simulink model "FAST"  (R2017b)
settings: Solver=FixedStepAuto  StartTime=0.0  StopTime=TMax  FixedStep=DT  RelTol=1e-3
values from neighbouring files (symbols this model uses):
  CertificationSettings = handles.CertificationSettings    [Certification.m]
  Control = handles.Control    [Certification.m]    (also in Linearization.m)
  dLP = ss(c2d(LP, Control.DT))    [ControllerDesign.m]
  dLP_IPC = ss(c2d(LP_IPC, Control.DT))    [ControllerDesign.m]
  dNotch = ss(c2d(Notch, Control.DT))    [ControllerDesign.m]
  Drivetrain = handles.Drivetrain    [Certification.m]    (also in Linearization.m)
  P_InitAngle = Control.Pitch.Max    [Certification.m]
  RPM_Init = 0    [Certification.m]
undefined symbols (not defined in the file or in its folder): AziPhase_offset_rev_1P, AziPhase_offset_rev_2P, DisableIPC_1P, DisableIPC_2P, DiscIntNeverNeededParam, OutList, strmatch, T_GenSpeedInit
libraries: simulink x5
(part 1 of 2)
settings Model: ExtModeTrigMode=oneshot  ExtModeArmWhenConnect=off  Creator=Hazim Namik  LastModifiedBy=sebastiaanmuld
settings DataIOCC: LimitDataPoints=on  SaveFormat=Array
settings OptimizationCC: BlockReduction=off  BooleanDataType=off  LifeSpan=inf
settings DebuggingCC: SaveWithParameterizedLinksMsg=none  UnderspecifiedInitializationDetection=Classic  MergeDetectMultiDrivingBlocksExec=none  SignalResolutionControl=TryResolveAllWithWarning  SFUnexpectedBacktrackingDiag=warning  SFNoUnconditionalDefaultTransitionDiag=warning  SFExecutionAtInitializationDiag=none
settings HardwareCC: ProdBitPerPointer=32  ProdBitPerSizeT=32  ProdBitPerPtrDiffT=32  ProdLargestAtomicFloat=None  ProdIntDivRoundTo=Undefined  ProdEndianess=Unspecified  ProdWordSize=32  ProdHWDeviceType=32-bit Generic  TargetUnknown=on
settings ModelReferenceCC: PropagateSignalLabelsOutOfModel=off
settings CodeAppCC: StateflowObjectComments=on
settings GRTTargetCC: TargetLangStandard=C89/C90 (ANSI)  GeneratePreprocessorConditionals=Disable all
settings ConfigComp: CovMetricSettings=dw  CovHtmlReporting=on  CovSaveCumulativeToWorkspaceVar=on  CovSaveSingleToWorkspaceVar=on  CovExternalEMLEnable=off

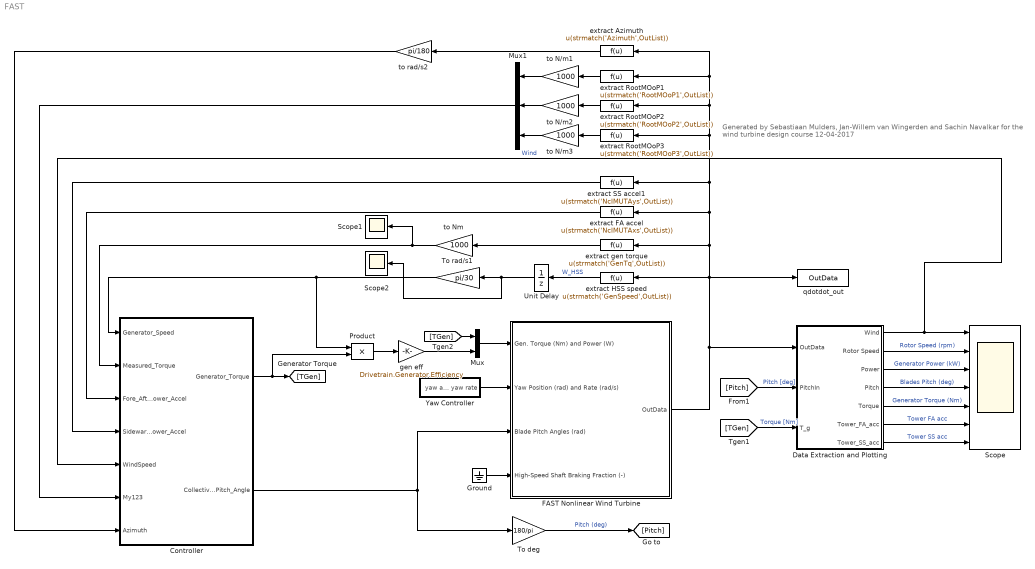
== system FAST ==
  note: Generated by Sebastiaan Mulders, Jan-Willem van Wingerden and Sachin Navalkar
      | for the wind turbine design course 12-04-2017
  Controller : Subsystem
  Data Extraction and Plotting : Subsystem
  FAST Nonlinear Wind Turbine : Subsystem  mask(FAST Nonlinear Wind Turbine){}
      mask help: This block contains the FAST S-Function.
      mask init:
      | clear FAST_SFunc
  Ground : Ground
  Mux : Mux  Inputs=2
  Mux1 : Mux  Inputs=3
  Product : Product  RndMeth=Zero
  Scope : Scope  NumInputPorts=7
      settings: Tag=Scope
  Scope1 : Scope
  Scope2 : Scope
  To deg : Gain  Gain=180/pi
  To rad/s1 : Gain  Gain=pi/30
  Unit Delay : UnitDelay  InitialCondition=RPM_Init*Drivetrain.Gearbox.Ratio  SampleTime=-1
  Yaw Controller : Subsystem
  extract Azimuth : Fcn  Expr=u(strmatch('Azimuth',OutList))
  extract FA accel : Fcn  Expr=u(strmatch('NcIMUTAxs',OutList))
  extract HSS speed : Fcn  Expr=u(strmatch('GenSpeed',OutList))
  extract RootMOoP1 : Fcn  Expr=u(strmatch('RootMOoP1',OutList))
  extract RootMOoP2 : Fcn  Expr=u(strmatch('RootMOoP2',OutList))
  extract RootMOoP3 : Fcn  Expr=u(strmatch('RootMOoP3',OutList))
  extract SS accel1 : Fcn  Expr=u(strmatch('NcIMUTAys',OutList))
  extract gen torque : Fcn  Expr=u(strmatch('GenTq',OutList))
  gen eff : Gain  Gain=Drivetrain.Generator.Efficiency
  qdotdot_out : ToWorkspace  VariableName=OutData  SampleTime=-1
      settings: Save2DSignal=2-D array (concatenate along first dimension)
  to N/m1 : Gain  Gain=1000
  to N/m2 : Gain  Gain=1000
  to N/m3 : Gain  Gain=1000
  to Nm : Gain  Gain=1000
  to rad/s2 : Gain  Gain=pi/180
  wires:
  Mux/1 -> FAST Nonlinear Wind Turbine/1(Gen. Torque (Nm) and Power (W))
  Yaw Controller/1(yaw and yaw rate) -> FAST Nonlinear Wind Turbine/2(Yaw Position (rad) and Rate (rad/s))
  extract HSS speed/1 -> Unit Delay/1  "W_HSS"
  To deg/1 -> [Pitch]  "Pitch (deg)"
  gen eff/1 -> Mux/2
  Product/1 -> gen eff/1
  To rad/s1/1 -> Product/1, Controller/1(Generator_Speed)
  Data Extraction and Plotting/3(Power) -> Scope/3  "Generator Power (kW)"
  [Pitch] -> Data Extraction and Plotting/2(PitchIn)  "Pitch [deg]"
  Data Extraction and Plotting/1(Wind) -> Controller/5(WindSpeed), Scope/1  "Wind"
  Data Extraction and Plotting/2(Rotor Speed) -> Scope/2  "Rotor Speed (rpm)"
  [TGen] -> Data Extraction and Plotting/3(T_g)  "Torque [Nm]"
  FAST Nonlinear Wind Turbine/1(OutData) -> extract Azimuth/1, extract RootMOoP1/1, extract RootMOoP2/1, extract RootMOoP3/1, extract SS accel1/1, extract FA accel/1, extract gen torque/1, extract HSS speed/1, qdotdot_out/1, Data Extraction and Plotting/1(OutData)
  Data Extraction and Plotting/4(Pitch) -> Scope/4  "Blades Pitch (deg)"
  Data Extraction and Plotting/5(Torque) -> Scope/5  "Generator Torque (Nm)"
  Unit Delay/1 -> Scope2/1, To rad/s1/1
  extract gen torque/1 -> to Nm/1
  to Nm/1 -> Scope1/1, Controller/2(Measured_Torque)
  Controller/1(Generator_Torque) -> Product/2, [TGen]
  Controller/2(Collective_Pitch_Angle) -> FAST Nonlinear Wind Turbine/3(Blade Pitch Angles (rad)), To deg/1
  extract FA accel/1 -> Controller/3(Fore_Aft_Tower_Accel)
  extract SS accel1/1 -> Controller/4(Sidewards_Tower_Accel)
  Data Extraction and Plotting/6(Tower_FA_acc) -> Scope/6  "Tower FA acc"
  Data Extraction and Plotting/7(Tower_SS_acc) -> Scope/7  "Tower SS acc"
  Ground/1 -> FAST Nonlinear Wind Turbine/4(High-Speed Shaft Braking Fraction (-))
  [TGen] -> Mux/1
  extract Azimuth/1 -> to rad/s2/1
  Mux1/1 -> Controller/6(My123)
  extract RootMOoP1/1 -> to N/m1/1
  extract RootMOoP2/1 -> to N/m2/1
  extract RootMOoP3/1 -> to N/m3/1
  to rad/s2/1 -> Controller/7(Azimuth)
  to N/m1/1 -> Mux1/1
  to N/m2/1 -> Mux1/2
  to N/m3/1 -> Mux1/3

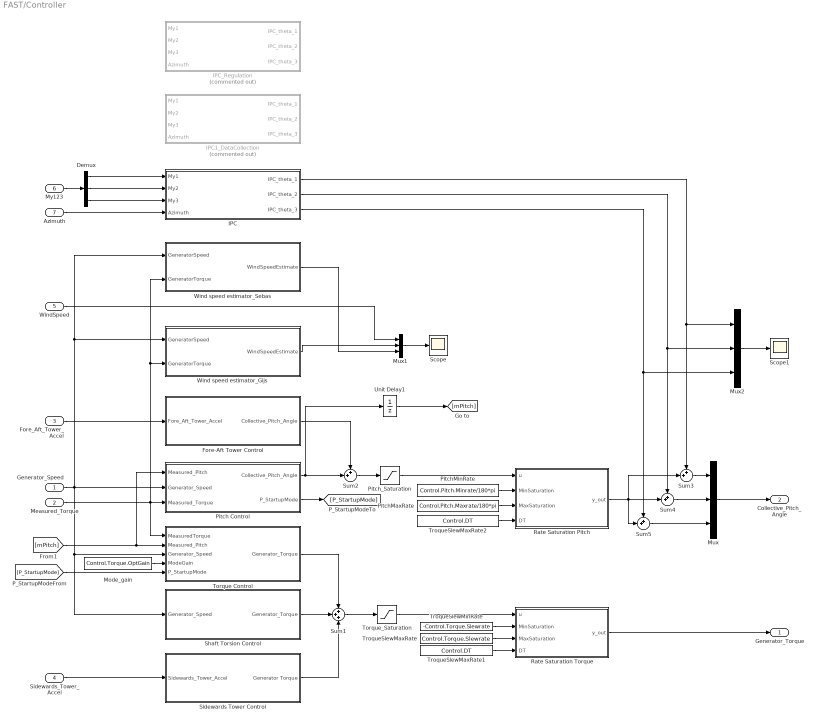
== system FAST/Controller ==
  Generator_Speed : Inport
  Measured_Torque : Inport  Port=2
  Fore_Aft_Tower_Accel : Inport  Port=3
  Sidewards_Tower_Accel : Inport  Port=4  PortDimensions=1
  WindSpeed : Inport  Port=5
  My123 : Inport  Port=6
  Azimuth : Inport  Port=7
  Demux : Demux  Outputs=3
  Fore-Aft Tower Control : Subsystem
  IPC : Subsystem
  IPC1_DataCollection : Subsystem  Commented=on
  IPC_Regulation : Subsystem  Commented=on
  Mode_gain : Constant  Value=Control.Torque.OptGain
  Mux : Mux  Inputs=3
  Mux1 : Mux  Inputs=3
  Mux2 : Mux  Inputs=3
  Pitch Control : Subsystem
  PitchMaxRate : Constant  Value=Control.Pitch.Maxrate/180*pi
  PitchMinRate : Constant  Value=Control.Pitch.Minrate/180*pi
  Pitch_Saturation : Saturate  UpperLimit=Control.Pitch.Max*pi/180  LowerLimit=Control.Pitch.Min*pi/180
  Rate Saturation Pitch : MATLAB Function  TreatAsAtomicUnit=on
  Rate Saturation Torque : MATLAB Function  TreatAsAtomicUnit=on
  Scope : Scope
  Scope1 : Scope
  Shaft Torsion Control : Subsystem
  Sidewards Tower Control : Subsystem
  Sum1 : Sum  Inputs=+++
  Sum{2..5} (4 alike) : Sum  Inputs=++|
  Torque Control : Subsystem
  Torque_Saturation : Saturate  UpperLimit=Control.Torque.Limit  LowerLimit=Control.Torque.Min
  TroqueSlewMaxRate : Constant  Value=Control.Torque.Slewrate
  TroqueSlewMaxRate1 : Constant  Value=Control.DT
  TroqueSlewMaxRate2 : Constant  Value=Control.DT
  TroqueSlewMinRate : Constant  Value=-Control.Torque.Slewrate
  Unit Delay1 : UnitDelay  InitialCondition=P_InitAngle*pi/180  SampleTime=-1
  Wind speed estimator_Gijs : Subsystem
  Wind speed estimator_Sebas : Subsystem
  Generator_Torque : Outport
  Collective_Pitch_Angle : Outport  Port=2  PortDimensions=3
  wires:
  Sidewards_Tower_Accel/1 -> Sidewards Tower Control/1(Sidewards_Tower_Accel)
  Fore_Aft_Tower_Accel/1 -> Fore-Aft Tower Control/1(Fore_Aft_Tower_Accel)
  Fore-Aft Tower Control/1(Collective_Pitch_Angle) -> Sum2/1
  Torque Control/1(Generator_Torque) -> Sum1/1
  Sidewards Tower Control/1(Generator Torque) -> Sum1/3
  [mPitch] -> Pitch Control/1(Measured_Pitch), Torque Control/2(Measured_Pitch)
  Measured_Torque/1 -> Wind speed estimator_Gijs/2(GeneratorTorque), Wind speed estimator_Sebas/2(GeneratorTorque), Torque Control/1(MeasuredTorque), Pitch Control/3(Measured_Torque)
  Shaft Torsion Control/1(Generator_Torque) -> Sum1/2
  Mode_gain/1 -> Torque Control/4(ModeGain)
  Sum1/1 -> Torque_Saturation/1
  Mux/1 -> Collective_Pitch_Angle/1
  Unit Delay1/1 -> [mPitch]
  Sum2/1 -> Pitch_Saturation/1
  Rate Saturation Pitch/1(y_out) -> Sum5/2, Sum4/2, Sum3/2
  PitchMinRate/1 -> Rate Saturation Pitch/2(MinSaturation)
  PitchMaxRate/1 -> Rate Saturation Pitch/3(MaxSaturation)
  Pitch_Saturation/1 -> Rate Saturation Pitch/1(u)
  Torque_Saturation/1 -> Rate Saturation Torque/1(u)
  TroqueSlewMinRate/1 -> Rate Saturation Torque/2(MinSaturation)
  TroqueSlewMaxRate/1 -> Rate Saturation Torque/3(MaxSaturation)
  Generator_Speed/1 -> Wind speed estimator_Sebas/1(GeneratorSpeed), Wind speed estimator_Gijs/1(GeneratorSpeed), Pitch Control/2(Generator_Speed), Torque Control/3(Generator_Speed), Shaft Torsion Control/1(Generator_Speed)
  [P_StartupMode] -> Torque Control/5(P_StartupMode)
  Pitch Control/2(P_StartupMode) -> [P_StartupMode]
  Pitch Control/1(Collective_Pitch_Angle) -> Sum2/2, Unit Delay1/1
  Rate Saturation Torque/1(y_out) -> Generator_Torque/1
  TroqueSlewMaxRate1/1 -> Rate Saturation Torque/4(DT)
  TroqueSlewMaxRate2/1 -> Rate Saturation Pitch/4(DT)
  Wind speed estimator_Gijs/1(WindSpeedEstimate) -> Mux1/2
  WindSpeed/1 -> Mux1/1
  Mux1/1 -> Scope/1
  My123/1 -> Demux/1
  Demux/1 -> IPC/1(My1)
  Demux/2 -> IPC/2(My2)
  Demux/3 -> IPC/3(My3)
  Azimuth/1 -> IPC/4(Azimuth)
  Sum3/1 -> Mux/1
  Sum4/1 -> Mux/2
  Sum5/1 -> Mux/3
  Mux2/1 -> Scope1/1
  IPC/1(IPC_theta_1) -> Mux2/1, Sum3/1
  IPC/2(IPC_theta_2) -> Mux2/2, Sum4/1
  IPC/3(IPC_theta_3) -> Sum5/1, Mux2/3
  Wind speed estimator_Sebas/1(WindSpeedEstimate) -> Mux1/3

== system FAST/Data Extraction and Plotting ==
  OutData : Inport
  PitchIn : Inport  Port=2
  T_g : Inport  Port=3
  Gain : Gain  Gain=1000
  Mux : Mux  Inputs=2
  extract Tower FA acc : Fcn  Expr=u(strmatch('NcIMUTAxs',OutList))
  extract Tower SS acc : Fcn  Expr=u(strmatch('NcIMUTAys',OutList))
  extract power : Fcn  Expr=u(strmatch('GenPwr',OutList))
  extract rotspeed : Fcn  Expr=u(strmatch('RotSpeed',OutList))
  extract w : Fcn  Expr=u(strmatch('Wind1VelX',OutList))
  extract w1 : Fcn  Expr=u(strmatch('GenTq',OutList))
  theta1 : ToWorkspace  VariableName=Tower_fa  SampleTime=-1
      settings: MaxDataPoints=Inf  Decimation=3
  theta2 : ToWorkspace  VariableName=GenPwr  SampleTime=-1
      settings: MaxDataPoints=Inf  Decimation=3
  theta3 : ToWorkspace  VariableName=wind  SampleTime=-1
      settings: MaxDataPoints=Inf  Decimation=3
  theta4 : ToWorkspace  VariableName=rotspeed  SampleTime=-1
      settings: MaxDataPoints=Inf  Decimation=3
  theta5 : ToWorkspace  VariableName=Tower_ss  SampleTime=-1
      settings: MaxDataPoints=Inf  Decimation=3
  theta6 : ToWorkspace  VariableName=pitch  SampleTime=-1
      settings: MaxDataPoints=Inf  Decimation=3
  theta7 : ToWorkspace  VariableName=Torque  SampleTime=-1
      settings: MaxDataPoints=Inf  Decimation=3
  Wind : Outport
  Rotor Speed : Outport  Port=2
  Power : Outport  Port=3
  Pitch : Outport  Port=4
  Torque : Outport  Port=5
  Tower_FA_acc : Outport  Port=6
  Tower_SS_acc : Outport  Port=7
  wires:
  extract w/1 -> Wind/1, theta3/1  "wind [m/s]"
  extract rotspeed/1 -> theta4/1, Rotor Speed/1  "rotspeed [rpm]"
  extract power/1 -> theta2/1, Power/1  "Power"
  PitchIn/1 -> theta6/1, Pitch/1
  T_g/1 -> Mux/1, theta7/1
  extract Tower FA acc/1 -> theta1/1, Tower_FA_acc/1  "Tower Fa acc"
  OutData/1 -> extract w/1, extract w1/1, extract rotspeed/1, extract Tower SS acc/1, extract Tower FA acc/1, extract power/1
  extract Tower SS acc/1 -> theta5/1, Tower_SS_acc/1  "Tower SS acc"
  extract w1/1 -> Gain/1
  Gain/1 -> Mux/2
  Mux/1 -> Torque/1

== system FAST/FAST Nonlinear Wind Turbine ==
  Gen. Torque (Nm) and Power (W) : Inport
  Yaw Position (rad) and Rate (rad/s) : Inport  Port=2
  Blade Pitch Angles (rad) : Inport  Port=3
  High-Speed Shaft Braking Fraction (-) : Inport  Port=4
  Mux1 : Mux
  S-Function : S-Function  FunctionName=FAST_SFunc  Parameters=FAST_InputFileName, TMax, 0  SFunctionDeploymentMode=off  EnableBusSupport=off
  Signal Specification1 : SignalSpecification  OutDataTypeStr=double  Dimensions=2
  Signal Specification2 : SignalSpecification  OutDataTypeStr=double  Dimensions=2
  OutData : Outport
  wires:
  Gen. Torque (Nm) and Power (W)/1 -> Signal Specification1/1
  S-Function/1 -> OutData/1
  Mux1/1 -> S-Function/1
  Blade Pitch Angles (rad)/1 -> Mux1/3
  Yaw Position (rad) and Rate (rad/s)/1 -> Signal Specification2/1
  Signal Specification1/1 -> Mux1/1
  Signal Specification2/1 -> Mux1/2
  High-Speed Shaft Braking Fraction (-)/1 -> Mux1/4

== system FAST/Yaw Controller ==
  Mux : Mux  Inputs=2
  Yaw Position : Constant  Value=0
  Yaw rate : Constant  Value=0
  yaw and yaw rate : Outport
  wires:
  Mux/1 -> yaw and yaw rate/1
  Yaw Position/1 -> Mux/1
  Yaw rate/1 -> Mux/2

== system FAST/Controller/Fore-Aft Tower Control ==
  note: Fore-Aft tower damping
  Fore_Aft_Tower_Accel : Inport
  Discrete-Time Integrator : DiscreteIntegrator  SampleTime=-1  ICPrevOutput=DiscIntNeverNeededParam  ICPrevScaledInput=DiscIntNeverNeededParam
  Gain : Gain  Gain=Control.ForeAft.Gain
  Pitch_Saturation : Saturate  UpperLimit=Control.ForeAft.MaxPitchAmplitude*pi/180  LowerLimit=-Control.ForeAft.MaxPitchAmplitude*pi/180
  Collective_Pitch_Angle : Outport
  wires:
  Fore_Aft_Tower_Accel/1 -> Discrete-Time Integrator/1
  Pitch_Saturation/1 -> Collective_Pitch_Angle/1
  Discrete-Time Integrator/1 -> Gain/1
  Gain/1 -> Pitch_Saturation/1

== system FAST/Controller/IPC ==
  My1 : Inport
  My2 : Inport  Port=2
  My3 : Inport  Port=3
  Azimuth : Inport  Port=4
  Constant : Constant
  DisableIPC : Constant  Value=DisableIPC_1P
  DisableIPC1 : Constant  Value=DisableIPC_2P
  Discrete-Time Integrator : DiscreteIntegrator  gainval=Ki_tilt_1P  ExternalReset=level  InitialConditionSetting=State (most efficient)  SampleTime=-1  LowerSaturationLimit=0  ICPrevOutput=DiscIntNeverNeededParam  ICPrevScaledInput=DiscIntNeverNeededParam
  Discrete-Time Integrator1 : DiscreteIntegrator  gainval=Ki_yaw_1P  ExternalReset=level  InitialConditionSetting=State (most efficient)  SampleTime=-1  LowerSaturationLimit=0  ICPrevOutput=DiscIntNeverNeededParam  ICPrevScaledInput=DiscIntNeverNeededParam
  Discrete-Time Integrator2 : DiscreteIntegrator  gainval=Ki_yaw_2P  ExternalReset=level  InitialConditionSetting=State (most efficient)  SampleTime=-1  ICPrevOutput=DiscIntNeverNeededParam  ICPrevScaledInput=DiscIntNeverNeededParam
  Discrete-Time Integrator3 : DiscreteIntegrator  gainval=Ki_tilt_2P  ExternalReset=level  InitialConditionSetting=State (most efficient)  SampleTime=-1  ICPrevOutput=DiscIntNeverNeededParam  ICPrevScaledInput=DiscIntNeverNeededParam
  Forward Coleman Transformation 1P : Subsystem
  Forward Coleman Transformation 3P : Subsystem
  Gain1 : Gain  Gain=pi/180
  Inverse Coleman Transformation 1P : Subsystem
  Inverse Coleman Transformation 3P : Subsystem
  Slider Gain : simulink/Math Operations/Slider Gain  gain=0.0  low=0  high=90
  Sum1 : Sum
  Sum2 : Sum
  Sum3 : Sum
  IPC_theta_1 : Outport
  IPC_theta_2 : Outport  Port=2
  IPC_theta_3 : Outport  Port=3
  wires:
  My1/1 -> Forward Coleman Transformation 3P/2(My_1), Forward Coleman Transformation 1P/2(My_1)
  My2/1 -> Forward Coleman Transformation 3P/3(My_2), Forward Coleman Transformation 1P/3(My_2)
  My3/1 -> Forward Coleman Transformation 3P/4(My_3), Forward Coleman Transformation 1P/4(My_3)
  Azimuth/1 -> Inverse Coleman Transformation 3P/1(Azimuth), Forward Coleman Transformation 3P/1(Azimuth), Inverse Coleman Transformation 1P/1(Azimuth), Forward Coleman Transformation 1P/1(Azimuth)
  Discrete-Time Integrator/1 -> Inverse Coleman Transformation 1P/2(theta_tilt)  "Ttilt"
  Discrete-Time Integrator1/1 -> Inverse Coleman Transformation 1P/3(theta_yaw)  "TYaw"
  Forward Coleman Transformation 3P/1(M_tilt) -> Discrete-Time Integrator3/1
  Forward Coleman Transformation 3P/2(M_yaw) -> Discrete-Time Integrator2/1
  Discrete-Time Integrator3/1 -> Inverse Coleman Transformation 3P/2(theta_tilt)
  Discrete-Time Integrator2/1 -> Inverse Coleman Transformation 3P/3(theta_yaw)
  Sum2/1 -> IPC_theta_1/1
  Sum1/1 -> IPC_theta_2/1
  Sum3/1 -> IPC_theta_3/1
  Inverse Coleman Transformation 3P/1(theta_1) -> Sum2/2
  Inverse Coleman Transformation 3P/2(theta_2) -> Sum1/2
  Inverse Coleman Transformation 3P/3(theta_3) -> Sum3/2
  Inverse Coleman Transformation 1P/3(theta_3) -> Sum3/1
  Inverse Coleman Transformation 1P/2(theta_2) -> Sum1/1
  Inverse Coleman Transformation 1P/1(theta_1) -> Sum2/1
  DisableIPC1/1 -> Discrete-Time Integrator2/2, Discrete-Time Integrator3/2
  Constant/1 -> Slider Gain/1
  Slider Gain/1 -> Gain1/1
  Gain1/1 -> Inverse Coleman Transformation 1P/4(PhaseOffset)
  DisableIPC/1 -> Discrete-Time Integrator1/2, Discrete-Time Integrator/2
  Forward Coleman Transformation 1P/1(M_tilt) -> Discrete-Time Integrator/1  "Mtilt"
  Forward Coleman Transformation 1P/2(M_yaw) -> Discrete-Time Integrator1/1  "Myaw"

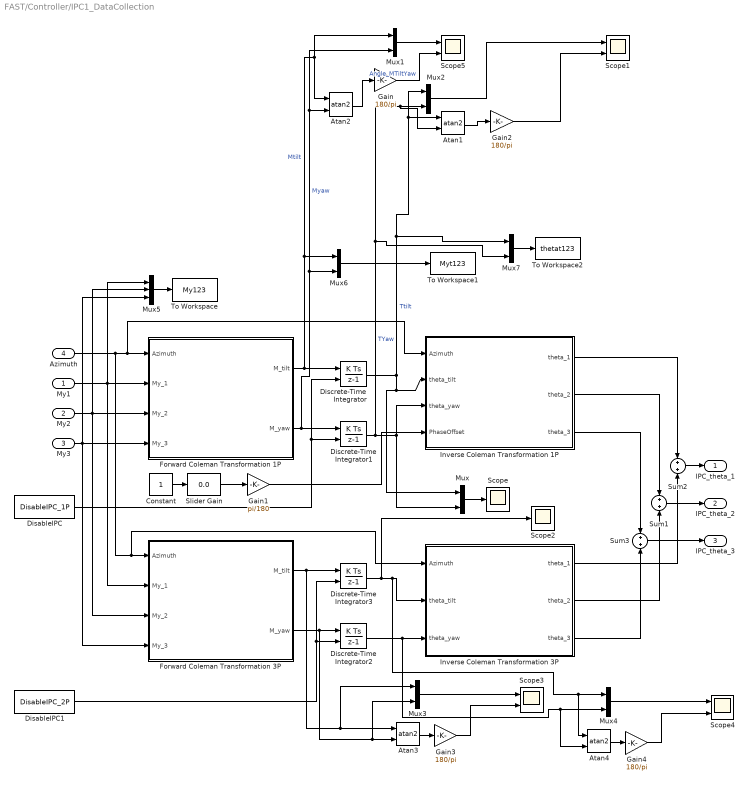
== system FAST/Controller/IPC1_DataCollection ==
  My1 : Inport
  My2 : Inport  Port=2
  My3 : Inport  Port=3
  Azimuth : Inport  Port=4
  Atan{1..4} (4 alike) : Trigonometry  Operator=atan2
  Constant : Constant
  DisableIPC : Constant  Value=DisableIPC_1P
  DisableIPC1 : Constant  Value=DisableIPC_2P
  Discrete-Time Integrator : DiscreteIntegrator  gainval=Ki_tilt_1P  ExternalReset=level  InitialConditionSetting=State (most efficient)  SampleTime=-1  ICPrevOutput=DiscIntNeverNeededParam  ICPrevScaledInput=DiscIntNeverNeededParam
  Discrete-Time Integrator1 : DiscreteIntegrator  gainval=Ki_yaw_1P  ExternalReset=level  InitialConditionSetting=State (most efficient)  SampleTime=-1  ICPrevOutput=DiscIntNeverNeededParam  ICPrevScaledInput=DiscIntNeverNeededParam
  Discrete-Time Integrator2 : DiscreteIntegrator  gainval=Ki_yaw_2P  ExternalReset=level  InitialConditionSetting=State (most efficient)  SampleTime=-1  ICPrevOutput=DiscIntNeverNeededParam  ICPrevScaledInput=DiscIntNeverNeededParam
  Discrete-Time Integrator3 : DiscreteIntegrator  gainval=Ki_tilt_2P  ExternalReset=level  InitialConditionSetting=State (most efficient)  SampleTime=-1  ICPrevOutput=DiscIntNeverNeededParam  ICPrevScaledInput=DiscIntNeverNeededParam
  Forward Coleman Transformation 1P : Subsystem
  Forward Coleman Transformation 3P : Subsystem
  Gain{,2..4} (4 alike) : Gain  Gain=180/pi
  Gain1 : Gain  Gain=pi/180
  Inverse Coleman Transformation 1P : Subsystem
  Inverse Coleman Transformation 3P : Subsystem
  Mux{,1..4,6..7} (7 alike) : Mux  Inputs=2
  Mux5 : Mux  Inputs=3
  Scope : Scope
  Scope{1,3..5} (4 alike) : Scope  NumInputPorts=2
  Scope2 : Scope
  Slider Gain : simulink/Math Operations/Slider Gain  gain=0.0  low=0  high=90
  Sum1 : Sum
  Sum2 : Sum
  Sum3 : Sum
  To Workspace : ToWorkspace  VariableName=My123  SaveFormat=Timeseries  SampleTime=-1
  To Workspace1 : ToWorkspace  VariableName=Myt123  SaveFormat=Timeseries  SampleTime=-1
  To Workspace2 : ToWorkspace  VariableName=thetat123  SaveFormat=Timeseries  SampleTime=-1
  IPC_theta_1 : Outport
  IPC_theta_2 : Outport  Port=2
  IPC_theta_3 : Outport  Port=3
  wires:
  Mux7/1 -> To Workspace2/1
  Mux6/1 -> To Workspace1/1
  Mux5/1 -> To Workspace/1
  Gain/1 -> Scope5/2  "Angle_MTiltYaw"
  Mux1/1 -> Scope5/1
  Gain4/1 -> Scope4/2
  Mux4/1 -> Scope4/1
  Atan4/1 -> Gain4/1
  Gain3/1 -> Scope3/2
  Mux3/1 -> Scope3/1
  Atan3/1 -> Gain3/1
  Gain2/1 -> Scope1/2
  Atan1/1 -> Gain2/1
  Mux2/1 -> Scope1/1
  Gain1/1 -> Inverse Coleman Transformation 1P/4(PhaseOffset)
  Slider Gain/1 -> Gain1/1
  Constant/1 -> Slider Gain/1
  Atan2/1 -> Gain/1
  DisableIPC1/1 -> Discrete-Time Integrator3/2, Discrete-Time Integrator2/2
  Inverse Coleman Transformation 1P/1(theta_1) -> Sum2/1
  Inverse Coleman Transformation 1P/2(theta_2) -> Sum1/1
  Inverse Coleman Transformation 1P/3(theta_3) -> Sum3/1
  Inverse Coleman Transformation 3P/3(theta_3) -> Sum3/2
  Inverse Coleman Transformation 3P/2(theta_2) -> Sum1/2
  Inverse Coleman Transformation 3P/1(theta_1) -> Sum2/2
  Sum3/1 -> IPC_theta_3/1
  Sum1/1 -> IPC_theta_2/1
  Sum2/1 -> IPC_theta_1/1
  Discrete-Time Integrator2/1 -> Inverse Coleman Transformation 3P/3(theta_yaw), Mux4/2, Atan4/2
  Discrete-Time Integrator3/1 -> Inverse Coleman Transformation 3P/2(theta_tilt), Mux4/1, Atan4/1, Scope2/1
  Forward Coleman Transformation 3P/2(M_yaw) -> Discrete-Time Integrator2/1, Atan3/2, Mux3/2
  Forward Coleman Transformation 3P/1(M_tilt) -> Discrete-Time Integrator3/1, Atan3/1, Mux3/1
  Mux/1 -> Scope/1
  DisableIPC/1 -> Discrete-Time Integrator/2, Discrete-Time Integrator1/2
  Discrete-Time Integrator1/1 -> Inverse Coleman Transformation 1P/3(theta_yaw), Mux/2, Mux2/2, Atan1/2, Mux7/2  "TYaw"
  Forward Coleman Transformation 1P/2(M_yaw) -> Discrete-Time Integrator1/1, Mux6/2, Mux1/2, Atan2/2  "Myaw"
  Forward Coleman Transformation 1P/1(M_tilt) -> Discrete-Time Integrator/1, Mux6/1, Mux1/1, Atan2/1  "Mtilt"
  Discrete-Time Integrator/1 -> Atan1/1, Mux2/1, Mux7/1, Inverse Coleman Transformation 1P/2(theta_tilt), Mux/1  "Ttilt"
  Azimuth/1 -> Forward Coleman Transformation 1P/1(Azimuth), Inverse Coleman Transformation 1P/1(Azimuth), Forward Coleman Transformation 3P/1(Azimuth), Inverse Coleman Transformation 3P/1(Azimuth)
  My3/1 -> Forward Coleman Transformation 1P/4(My_3), Forward Coleman Transformation 3P/4(My_3), Mux5/3
  My2/1 -> Forward Coleman Transformation 1P/3(My_2), Forward Coleman Transformation 3P/3(My_2), Mux5/2
  My1/1 -> Forward Coleman Transformation 1P/2(My_1), Forward Coleman Transformation 3P/2(My_1), Mux5/1

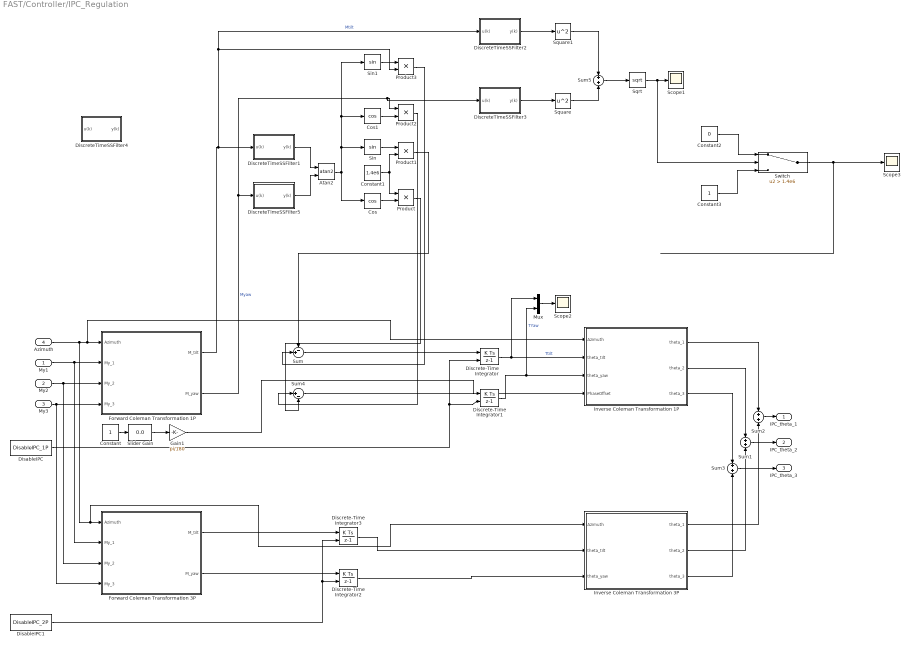
== system FAST/Controller/IPC_Regulation ==
  My1 : Inport
  My2 : Inport  Port=2
  My3 : Inport  Port=3
  Azimuth : Inport  Port=4
  Atan2 : Trigonometry  Operator=atan2
  Constant : Constant
  Constant1 : Constant  Value=1.4e6
  Constant2 : Constant  Value=0
  Constant3 : Constant
  Cos : Trigonometry  Operator=cos
  Cos1 : Trigonometry  Operator=cos
  DisableIPC : Constant  Value=DisableIPC_1P
  DisableIPC1 : Constant  Value=DisableIPC_2P
  Discrete-Time Integrator : DiscreteIntegrator  gainval=Ki_tilt_1P  ExternalReset=level  InitialConditionSetting=State (most efficient)  SampleTime=-1  LowerSaturationLimit=0  ICPrevOutput=DiscIntNeverNeededParam  ICPrevScaledInput=DiscIntNeverNeededParam
  Discrete-Time Integrator1 : DiscreteIntegrator  gainval=Ki_yaw_1P  ExternalReset=level  InitialConditionSetting=State (most efficient)  SampleTime=-1  LowerSaturationLimit=0  ICPrevOutput=DiscIntNeverNeededParam  ICPrevScaledInput=DiscIntNeverNeededParam
  Discrete-Time Integrator2 : DiscreteIntegrator  gainval=Ki_yaw_2P  ExternalReset=level  InitialConditionSetting=State (most efficient)  SampleTime=-1  ICPrevOutput=DiscIntNeverNeededParam  ICPrevScaledInput=DiscIntNeverNeededParam
  Discrete-Time Integrator3 : DiscreteIntegrator  gainval=Ki_tilt_2P  ExternalReset=level  InitialConditionSetting=State (most efficient)  SampleTime=-1  ICPrevOutput=DiscIntNeverNeededParam  ICPrevScaledInput=DiscIntNeverNeededParam
  DiscreteTimeSSFilter1 : Subsystem
  DiscreteTimeSSFilter2 : Subsystem
  DiscreteTimeSSFilter3 : Subsystem
  DiscreteTimeSSFilter4 : Subsystem
  DiscreteTimeSSFilter5 : Subsystem
  Forward Coleman Transformation 1P : Subsystem
  Forward Coleman Transformation 3P : Subsystem
  Gain1 : Gain  Gain=pi/180
  Inverse Coleman Transformation 1P : Subsystem
  Inverse Coleman Transformation 3P : Subsystem
  Mux : Mux  Inputs=2
  Product{,1..3} (4 alike) : Product
  Scope1 : Scope
  Scope2 : Scope
  Scope3 : Scope
  Sin : Trigonometry
  Sin1 : Trigonometry
  Slider Gain : simulink/Math Operations/Slider Gain  gain=0.0  low=0  high=90
  Sqrt : Sqrt  SaturateOnIntegerOverflow=on
  Square : Math  Operator=square  RndMeth=Zero  SaturateOnIntegerOverflow=on
  Square1 : Math  Operator=square  RndMeth=Zero  SaturateOnIntegerOverflow=on
  Sum : Sum  Inputs=-+|
  Sum{1..3,5} (4 alike) : Sum
  Sum4 : Sum  Inputs=|+-
  Switch : Switch  Criteria=u2 > Threshold  Threshold=1.4e6
  IPC_theta_1 : Outport
  IPC_theta_2 : Outport  Port=2
  IPC_theta_3 : Outport  Port=3
  wires:
  DisableIPC/1 -> Discrete-Time Integrator/2, Discrete-Time Integrator1/2
  DiscreteTimeSSFilter2/1(y(k)) -> Square1/1
  DiscreteTimeSSFilter3/1(y(k)) -> Square/1
  Product3/1 -> Sum/2
  Product1/1 -> Sum/1
  Product2/1 -> Sum4/1
  Product/1 -> Sum4/2
  Switch/1 -> Scope3/1
  Constant3/1 -> Switch/3
  Constant2/1 -> Switch/1
  Mux/1 -> Scope2/1
  Sin1/1 -> Product3/1
  Cos1/1 -> Product2/2
  Cos/1 -> Product/2
  Constant1/1 -> Product1/2, Product/1
  Sum4/1 -> Discrete-Time Integrator1/1
  Sum/1 -> Discrete-Time Integrator/1
  Sqrt/1 -> Scope1/1, Switch/2
  Sum5/1 -> Sqrt/1
  Square/1 -> Sum5/2
  Square1/1 -> Sum5/1
  Sin/1 -> Product1/1
  Atan2/1 -> Sin/1, Sin1/1, Cos1/1, Cos/1
  DiscreteTimeSSFilter5/1(y(k)) -> Atan2/2
  DiscreteTimeSSFilter1/1(y(k)) -> Atan2/1
  Forward Coleman Transformation 1P/1(M_tilt) -> DiscreteTimeSSFilter2/1(u(k)), Product3/2, DiscreteTimeSSFilter1/1(u(k))  "Mtilt"
  Gain1/1 -> Inverse Coleman Transformation 1P/4(PhaseOffset)
  Slider Gain/1 -> Gain1/1
  Constant/1 -> Slider Gain/1
  DisableIPC1/1 -> Discrete-Time Integrator3/2, Discrete-Time Integrator2/2
  Inverse Coleman Transformation 1P/1(theta_1) -> Sum2/1
  Inverse Coleman Transformation 1P/2(theta_2) -> Sum1/1
  Inverse Coleman Transformation 1P/3(theta_3) -> Sum3/1
  Inverse Coleman Transformation 3P/3(theta_3) -> Sum3/2
  Inverse Coleman Transformation 3P/2(theta_2) -> Sum1/2
  Inverse Coleman Transformation 3P/1(theta_1) -> Sum2/2
  Sum3/1 -> IPC_theta_3/1
  Sum1/1 -> IPC_theta_2/1
  Sum2/1 -> IPC_theta_1/1
  Discrete-Time Integrator2/1 -> Inverse Coleman Transformation 3P/3(theta_yaw)
  Discrete-Time Integrator3/1 -> Inverse Coleman Transformation 3P/2(theta_tilt)
  Forward Coleman Transformation 3P/2(M_yaw) -> Discrete-Time Integrator2/1
  Forward Coleman Transformation 3P/1(M_tilt) -> Discrete-Time Integrator3/1
  Discrete-Time Integrator1/1 -> Inverse Coleman Transformation 1P/3(theta_yaw), Mux/2  "TYaw"
  Forward Coleman Transformation 1P/2(M_yaw) -> Product2/1, DiscreteTimeSSFilter3/1(u(k)), DiscreteTimeSSFilter5/1(u(k))  "Myaw"
  Discrete-Time Integrator/1 -> Inverse Coleman Transformation 1P/2(theta_tilt), Mux/1  "Ttilt"
  Azimuth/1 -> Forward Coleman Transformation 1P/1(Azimuth), Inverse Coleman Transformation 1P/1(Azimuth), Forward Coleman Transformation 3P/1(Azimuth), Inverse Coleman Transformation 3P/1(Azimuth)
  My3/1 -> Forward Coleman Transformation 1P/4(My_3), Forward Coleman Transformation 3P/4(My_3)
  My2/1 -> Forward Coleman Transformation 1P/3(My_2), Forward Coleman Transformation 3P/3(My_2)
  My1/1 -> Forward Coleman Transformation 1P/2(My_1), Forward Coleman Transformation 3P/2(My_1)

== system FAST/Controller/Pitch Control ==
  Measured_Pitch : Inport
  Generator_Speed : Inport  Port=2
  Measured_Torque : Inport  Port=3
  Clock : Clock
  DT : Constant  Value=Control.DT
  DemandedTorque : Constant  Value=Control.Torque.Demanded
  EventActionTime : Constant  Value=CertificationSettings.Mode.Actiontime
  EventType : Constant  Value=CertificationSettings.Mode.Type
  GainScheduler : Subsystem
  GearboxRatio : Constant  Value=Drivetrain.Gearbox.Ratio
  InitialPitchAngle : Constant  Value=P_InitAngle
  Lowpass Filter : Subsystem
  MinMaxPitch : Constant  Value=[Control.Pitch.Fine Control.Pitch.Max]
  MinMaxPitchRate : Constant  Value=[Control.Pitch.Minrate Control.Pitch.Maxrate]
  P_StartupPitch : Constant  Value=Control.Pitch.StartupPitch
  P_StartupPitchRate : Constant  Value=Control.Pitch.StartupPitchRate
  P_StartupSpeed : Constant  Value=Control.Pitch.StartupSpeed
  PitchControl : MATLAB Function  TreatAsAtomicUnit=on
  Scope : Scope
  Scope1 : Scope
  SpeedC : Constant  Value=Control.Torque.SpeedC*pi/30
  SpeedC_2 : Constant  Value=Control.Torque.SpeedC
  Sum : Sum  Inputs=|+-
  Collective_Pitch_Angle : Outport
  P_StartupMode : Outport  Port=2
  wires:
  MinMaxPitch/1 -> PitchControl/7(MinMaxPitch)
  MinMaxPitchRate/1 -> PitchControl/8(MinMaxPitchRate)
  PitchControl/1(BladePitch) -> Scope/1, Collective_Pitch_Angle/1
  Measured_Torque/1 -> PitchControl/3(MeasuredTorque)
  SpeedC/1 -> Sum/1
  Generator_Speed/1 -> PitchControl/2(GeneratorSpeed), Sum/2
  Sum/1 -> Scope1/1, Lowpass Filter/1(Input)
  Lowpass Filter/1(Output) -> PitchControl/1(GeneratorSpeedError)
  PitchControl/2(P_LowRateModeOut) -> P_StartupMode/1
  DT/1 -> PitchControl/9(DT)
  P_StartupPitch/1 -> PitchControl/11(P_StartupPitch)
  InitialPitchAngle/1 -> PitchControl/10(P_InitAngle)
  GearboxRatio/1 -> PitchControl/12(GearboxRatio)
  P_StartupSpeed/1 -> PitchControl/13(P_StartUpSpeed)
  P_StartupPitchRate/1 -> PitchControl/14(P_StartupPitchRate)
  SpeedC_2/1 -> PitchControl/15(omega_C)
  DemandedTorque/1 -> PitchControl/16(Demanded_torque)
  Measured_Pitch/1 -> PitchControl/4(MeasuredPitch), GainScheduler/1(MeasuredPitch)
  EventType/1 -> PitchControl/18(Event)
  Clock/1 -> PitchControl/17(Clock)
  EventActionTime/1 -> PitchControl/19(EventTime)
  GainScheduler/1(Kp) -> PitchControl/5(KP)
  GainScheduler/2(Ki) -> PitchControl/6(KI)

== system FAST/Controller/Shaft Torsion Control ==
  Generator_Speed : Inport
  Gain : Gain  Gain=0
  Generator_Torque : Outport
  wires:
  Generator_Speed/1 -> Gain/1
  Gain/1 -> Generator_Torque/1

== system FAST/Controller/Sidewards Tower Control ==
  Sidewards_Tower_Accel : Inport
  Gain : Gain  Gain=0
  Generator Torque : Outport
  wires:
  Sidewards_Tower_Accel/1 -> Gain/1
  Gain/1 -> Generator Torque/1

== system FAST/Controller/Torque Control ==
  MeasuredTorque : Inport
  Measured_Pitch : Inport  Port=2
  Generator_Speed : Inport  Port=3
  ModeGain : Inport  Port=4
  P_StartupMode : Inport  Port=5
  DT : Constant  Value=Control.DT
  Low-pass filter : Subsystem
  Torque Controller set points : Constant  Value=[Control.Torque.SpeedA Control.Torque.SpeedB Control.Torque.SpeedB2 Control.Torque.SpeedC]
  Torque Controller set points1 : Constant  Value=Control.Torque.Demanded
  Torque Controller set points2 : Constant  Value=Control.Pitch.Fine
  Torque Controller set points3 : Constant  Value=Control.Torque.Min
  Torque Controller set points4 : Constant  Value=[-4200 -2100]
  TorqueController : MATLAB Function  TreatAsAtomicUnit=on
  Generator_Torque : Outport
  wires:
  Generator_Speed/1 -> Low-pass filter/1(Input)
  TorqueController/1(GeneratorTorqueDemand) -> Generator_Torque/1
  Measured_Pitch/1 -> TorqueController/3(MeasuredPitch)
  ModeGain/1 -> TorqueController/4(Control_Torque_OptGain)
  Torque Controller set points/1 -> TorqueController/5(omega_ABCD)
  P_StartupMode/1 -> TorqueController/6(P_StartupMode)
  Low-pass filter/1(Output) -> TorqueController/2(MeasuredGeneratorSpeed)
  Torque Controller set points3/1 -> TorqueController/9(T_MinTorque)
  Torque Controller set points2/1 -> TorqueController/8(Pitch_Fine)
  Torque Controller set points1/1 -> TorqueController/7(Torque_Demanded)
  Torque Controller set points4/1 -> TorqueController/10(KpKi_TorqueControl)
  MeasuredTorque/1 -> TorqueController/1(MeasuredTorque)
  DT/1 -> TorqueController/11(DT)

== system FAST/Controller/Wind speed estimator_Gijs ==
  GeneratorSpeed : Inport
  GeneratorTorque : Inport  Port=2
  Discrete Derivative : simulink/Discrete/Discrete Derivative  gainval=1.0  ICPrevScaledInput=0.0  OutMin=[]  OutMax=[]  OutDataType=fixdt(1, 16)  OutScaling=2^-10  DoSatur=off
  Divide : Product  Inputs=/*
  Divide1 : Product  Inputs=*/
  G : Gain  Gain=Drivetrain.Gearbox.Ratio
  G1 : Gain  Gain=Drivetrain.Gearbox.Ratio
  G_times_Irotor : Gain  Gain=38677040.613*Drivetrain.Gearbox.Ratio
  Lamda(Fq) : Lookup_n-D  NumberOfTableDimensions=1  BreakpointsForDimension1=CQ_lambda(3,end-24:-1:31)  Table=CQ_lambda(1,end-24:-1:31)  InternalRulePriority=Speed  RndMeth=Simplest  InputSameDT=on
  Lowpass Filter : Subsystem
  Mux : Mux  Inputs=3
  Mux1 : Mux  Inputs=2
  RotorConstant : Gain  Gain=2/(1.225*pi*Blade.Radius(end)^5)
  Scope{,1..3} (4 alike) : Scope
  Square : Math  Operator=square  RndMeth=Zero  SaturateOnIntegerOverflow=on
  Sum : Sum  Inputs=|++
  omega_times_R : Gain  Gain=Blade.Radius(end)/Drivetrain.Gearbox.Ratio
  WindSpeedEstimate : Outport
  wires:
  Discrete Derivative/1 -> Mux/3, G_times_Irotor/1
  GeneratorTorque/1 -> G/1
  Sum/1 -> RotorConstant/1
  RotorConstant/1 -> Divide/2
  Square/1 -> Divide/1
  Divide/1 -> Lamda(Fq)/1
  Lamda(Fq)/1 -> Scope1/1, Divide1/2
  omega_times_R/1 -> Scope2/1, Divide1/1
  Mux/1 -> Scope/1
  GeneratorSpeed/1 -> Lowpass Filter/1(Input), Mux/1
  G_times_Irotor/1 -> Mux1/1, Sum/1
  Mux1/1 -> Scope3/1
  Lowpass Filter/1(Output) -> omega_times_R/1, G1/1, Mux/2, Discrete Derivative/1
  G/1 -> Mux1/2, Sum/2
  G1/1 -> Square/1
  Divide1/1 -> WindSpeedEstimate/1

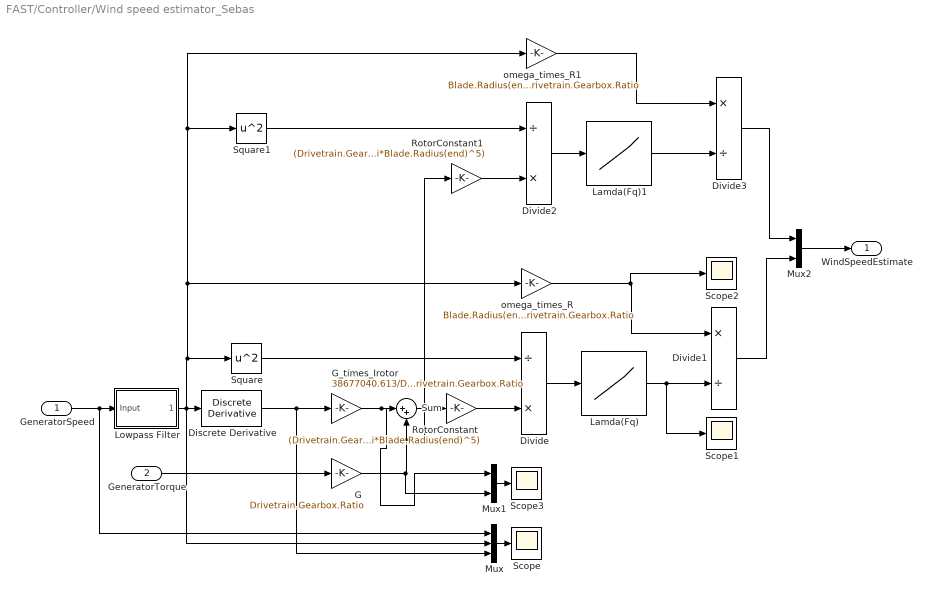
== system FAST/Controller/Wind speed estimator_Sebas ==
  GeneratorSpeed : Inport
  GeneratorTorque : Inport  Port=2
  Discrete Derivative : simulink/Discrete/Discrete Derivative  gainval=1.0  ICPrevScaledInput=0.0  OutMin=[]  OutMax=[]  OutDataType=fixdt(1, 16)  OutScaling=2^-10  DoSatur=off
  Divide : Product  Inputs=/*
  Divide1 : Product  Inputs=*/
  Divide2 : Product  Inputs=/*
  Divide3 : Product  Inputs=*/
  G : Gain  Gain=Drivetrain.Gearbox.Ratio
  G_times_Irotor : Gain  Gain=38677040.613/Drivetrain.Gearbox.Ratio
  Lamda(Fq) : Lookup_n-D  NumberOfTableDimensions=1  BreakpointsForDimension1=CQ_lambda(3,end-24:-1:31)  Table=CQ_lambda(1,end-24:-1:31)  InternalRulePriority=Speed  RndMeth=Simplest  InputSameDT=on
  Lamda(Fq)1 : Lookup_n-D  NumberOfTableDimensions=1  BreakpointsForDimension1=CQ_lambda(3,end-24:-1:31)  Table=CQ_lambda(1,end-24:-1:31)  InternalRulePriority=Speed  RndMeth=Simplest  InputSameDT=on
  Lowpass Filter : Subsystem
  Mux : Mux  Inputs=3
  Mux1 : Mux  Inputs=2
  Mux2 : Mux  Inputs=2
  RotorConstant : Gain  Gain=(Drivetrain.Gearbox.Ratio)^2/(1/2*1.225*pi*Blade.Radius(end)^5)
  RotorConstant1 : Gain  Gain=(Drivetrain.Gearbox.Ratio)^2/(1/2*1.225*pi*Blade.Radius(end)^5)
  Scope{,1..3} (4 alike) : Scope
  Square : Math  Operator=square  RndMeth=Zero  SaturateOnIntegerOverflow=on
  Square1 : Math  Operator=square  RndMeth=Zero  SaturateOnIntegerOverflow=on
  Sum : Sum  Inputs=|++
  omega_times_R : Gain  Gain=Blade.Radius(end)/Drivetrain.Gearbox.Ratio
  omega_times_R1 : Gain  Gain=Blade.Radius(end)/Drivetrain.Gearbox.Ratio
  WindSpeedEstimate : Outport
  wires:
  Divide1/1 -> Mux2/2
  Mux2/1 -> WindSpeedEstimate/1
  RotorConstant1/1 -> Divide2/2
  G/1 -> Sum/2, RotorConstant1/1, Mux1/2
  Square1/1 -> Divide2/1
  Divide2/1 -> Lamda(Fq)1/1
  Lamda(Fq)1/1 -> Divide3/2
  Divide3/1 -> Mux2/1
  omega_times_R1/1 -> Divide3/1
  Lowpass Filter/1(Output) -> Discrete Derivative/1, Square/1, omega_times_R/1, omega_times_R1/1, Square1/1, Mux/2
  Mux1/1 -> Scope3/1
  G_times_Irotor/1 -> Sum/1, Mux1/1
  GeneratorSpeed/1 -> Lowpass Filter/1(Input), Mux/1
  Mux/1 -> Scope/1
  omega_times_R/1 -> Divide1/1, Scope2/1
  Lamda(Fq)/1 -> Divide1/2, Scope1/1
  Divide/1 -> Lamda(Fq)/1
  Square/1 -> Divide/1
  RotorConstant/1 -> Divide/2
  Sum/1 -> RotorConstant/1
  GeneratorTorque/1 -> G/1
  Discrete Derivative/1 -> G_times_Irotor/1, Mux/3

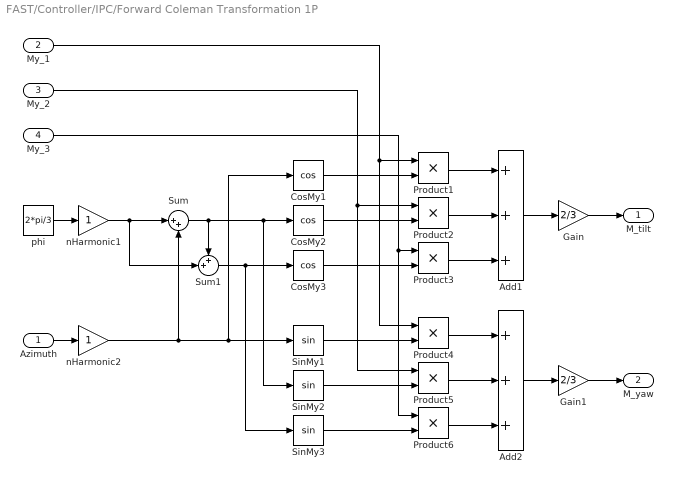
== system FAST/Controller/IPC/Forward Coleman Transformation 1P ==
  Azimuth : Inport
  My_1 : Inport  Port=2
  My_2 : Inport  Port=3
  My_3 : Inport  Port=4
  Add1 : Sum  Inputs=+++
  Add2 : Sum  Inputs=+++
  CosMy1 : Trigonometry  Operator=cos
  CosMy2 : Trigonometry  Operator=cos
  CosMy3 : Trigonometry  Operator=cos
  Gain : Gain  Gain=2/3
  Gain1 : Gain  Gain=2/3
  Product{1..6} (6 alike) : Product  RndMeth=Zero
  SinMy1 : Trigonometry
  SinMy2 : Trigonometry
  SinMy3 : Trigonometry
  Sum : Sum  Inputs=|++
  Sum1 : Sum  Inputs=++|
  nHarmonic1 : Gain
  nHarmonic2 : Gain
  phi : Constant  Value=2*pi/3
  M_tilt : Outport
  M_yaw : Outport  Port=2
  wires:
  Gain1/1 -> M_yaw/1
  Gain/1 -> M_tilt/1
  Product6/1 -> Add2/3
  SinMy3/1 -> Product6/2
  CosMy3/1 -> Product3/2
  My_3/1 -> Product3/1, Product6/1
  Product3/1 -> Add1/3
  Sum1/1 -> CosMy3/1, SinMy3/1
  Add2/1 -> Gain1/1
  Add1/1 -> Gain/1
  Product5/1 -> Add2/2
  Product4/1 -> Add2/1
  Product2/1 -> Add1/2
  Product1/1 -> Add1/1
  My_2/1 -> Product2/1, Product5/1
  My_1/1 -> Product1/1, Product4/1
  Sum/1 -> SinMy2/1, CosMy2/1, Sum1/1
  SinMy2/1 -> Product5/2
  SinMy1/1 -> Product4/2
  CosMy2/1 -> Product2/2
  CosMy1/1 -> Product1/2
  Azimuth/1 -> nHarmonic2/1
  phi/1 -> nHarmonic1/1
  nHarmonic1/1 -> Sum/1, Sum1/2
  nHarmonic2/1 -> SinMy1/1, CosMy1/1, Sum/2

== system FAST/Controller/IPC/Forward Coleman Transformation 3P ==
  Azimuth : Inport
  My_1 : Inport  Port=2
  My_2 : Inport  Port=3
  My_3 : Inport  Port=4
  Add1 : Sum  Inputs=+++
  Add2 : Sum  Inputs=+++
  CosMy1 : Trigonometry  Operator=cos
  CosMy2 : Trigonometry  Operator=cos
  CosMy3 : Trigonometry  Operator=cos
  Gain : Gain  Gain=2/3
  Gain1 : Gain  Gain=2/3
  Product{1..6} (6 alike) : Product  RndMeth=Zero
  SinMy1 : Trigonometry
  SinMy2 : Trigonometry
  SinMy3 : Trigonometry
  Sum : Sum  Inputs=|++
  Sum1 : Sum  Inputs=++|
  nHarmonic : Gain  Gain=3
  nHarmonic1 : Gain  Gain=3
  phi : Constant  Value=2*pi/3
  M_tilt : Outport
  M_yaw : Outport  Port=2
  wires:
  phi/1 -> nHarmonic/1
  Azimuth/1 -> nHarmonic1/1
  CosMy1/1 -> Product1/2
  CosMy2/1 -> Product2/2
  SinMy1/1 -> Product4/2
  SinMy2/1 -> Product5/2
  Sum/1 -> Sum1/1, CosMy2/1, SinMy2/1
  My_1/1 -> Product4/1, Product1/1
  My_2/1 -> Product5/1, Product2/1
  Product1/1 -> Add1/1
  Product2/1 -> Add1/2
  Product4/1 -> Add2/1
  Product5/1 -> Add2/2
  Add1/1 -> Gain/1
  Add2/1 -> Gain1/1
  Sum1/1 -> SinMy3/1, CosMy3/1
  Product3/1 -> Add1/3
  My_3/1 -> Product6/1, Product3/1
  CosMy3/1 -> Product3/2
  SinMy3/1 -> Product6/2
  Product6/1 -> Add2/3
  Gain/1 -> M_tilt/1
  Gain1/1 -> M_yaw/1
  nHarmonic/1 -> Sum1/2, Sum/1
  nHarmonic1/1 -> Sum/2, CosMy1/1, SinMy1/1

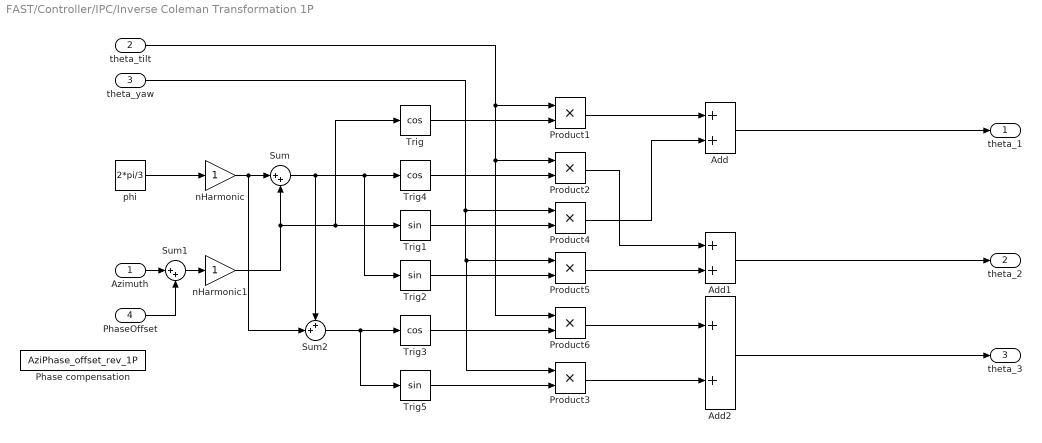
== system FAST/Controller/IPC/Inverse Coleman Transformation 1P ==
  Azimuth : Inport
  theta_tilt : Inport  Port=2
  theta_yaw : Inport  Port=3
  PhaseOffset : Inport  Port=4
  Add : Sum
  Add1 : Sum
  Add2 : Sum
  Phase compensation : Constant  Value=AziPhase_offset_rev_1P
  Product{1..6} (6 alike) : Product  RndMeth=Zero
  Sum : Sum  Inputs=|++
  Sum1 : Sum  Inputs=|++
  Sum2 : Sum  Inputs=++|
  Trig : Trigonometry  Operator=cos
  Trig1 : Trigonometry
  Trig2 : Trigonometry
  Trig3 : Trigonometry  Operator=cos
  Trig4 : Trigonometry  Operator=cos
  Trig5 : Trigonometry
  nHarmonic : Gain
  nHarmonic1 : Gain
  phi : Constant  Value=2*pi/3
  theta_1 : Outport
  theta_2 : Outport  Port=2
  theta_3 : Outport  Port=3
  wires:
  phi/1 -> nHarmonic/1
  nHarmonic1/1 -> Trig/1, Trig1/1, Sum/2
  Sum/1 -> Sum2/1, Trig4/1, Trig2/1
  Trig/1 -> Product1/2
  Trig4/1 -> Product2/2
  Trig1/1 -> Product4/2
  Trig2/1 -> Product5/2
  theta_tilt/1 -> Product1/1, Product6/1, Product2/1
  theta_yaw/1 -> Product3/1, Product5/1, Product4/1
  Product4/1 -> Add/2
  Product1/1 -> Add/1
  Product2/1 -> Add1/1
  Product5/1 -> Add1/2
  PhaseOffset/1 -> Sum1/2
  Product6/1 -> Add2/1
  Product3/1 -> Add2/2
  Sum2/1 -> Trig5/1, Trig3/1
  Trig3/1 -> Product6/2
  Trig5/1 -> Product3/2
  Add/1 -> theta_1/1
  Add1/1 -> theta_2/1
  Add2/1 -> theta_3/1
  nHarmonic/1 -> Sum2/2, Sum/1
  Azimuth/1 -> Sum1/1
  Sum1/1 -> nHarmonic1/1

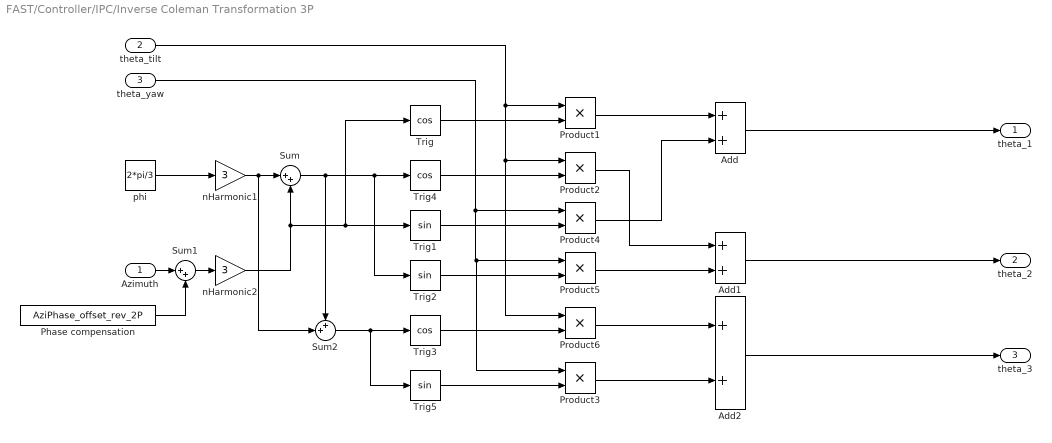
== system FAST/Controller/IPC/Inverse Coleman Transformation 3P ==
  Azimuth : Inport
  theta_tilt : Inport  Port=2
  theta_yaw : Inport  Port=3
  Add : Sum
  Add1 : Sum
  Add2 : Sum
  Phase compensation : Constant  Value=AziPhase_offset_rev_2P
  Product{1..6} (6 alike) : Product  RndMeth=Zero
  Sum : Sum  Inputs=|++
  Sum1 : Sum  Inputs=|++
  Sum2 : Sum  Inputs=++|
  Trig : Trigonometry  Operator=cos
  Trig1 : Trigonometry
  Trig2 : Trigonometry
  Trig3 : Trigonometry  Operator=cos
  Trig4 : Trigonometry  Operator=cos
  Trig5 : Trigonometry
  nHarmonic1 : Gain  Gain=3
  nHarmonic2 : Gain  Gain=3
  phi : Constant  Value=2*pi/3
  theta_1 : Outport
  theta_2 : Outport  Port=2
  theta_3 : Outport  Port=3
  wires:
  Add2/1 -> theta_3/1
  Add1/1 -> theta_2/1
  Add/1 -> theta_1/1
  Trig5/1 -> Product3/2
  Trig3/1 -> Product6/2
  Sum2/1 -> Trig3/1, Trig5/1
  Product3/1 -> Add2/2
  Product6/1 -> Add2/1
  Phase compensation/1 -> Sum1/2
  Product5/1 -> Add1/2
  Product2/1 -> Add1/1
  Product1/1 -> Add/1
  Product4/1 -> Add/2
  theta_yaw/1 -> Product4/1, Product5/1, Product3/1
  theta_tilt/1 -> Product2/1, Product6/1, Product1/1
  Trig2/1 -> Product5/2
  Trig1/1 -> Product4/2
  Trig4/1 -> Product2/2
  Trig/1 -> Product1/2
  Sum/1 -> Trig2/1, Trig4/1, Sum2/1
  Sum1/1 -> nHarmonic2/1
  phi/1 -> nHarmonic1/1
  nHarmonic1/1 -> Sum/1, Sum2/2
  Azimuth/1 -> Sum1/1
  nHarmonic2/1 -> Sum/2, Trig1/1, Trig/1

== system FAST/Controller/IPC1_DataCollection/Forward Coleman Transformation 1P ==
  Azimuth : Inport
  My_1 : Inport  Port=2
  My_2 : Inport  Port=3
  My_3 : Inport  Port=4
  Add1 : Sum  Inputs=+++
  Add2 : Sum  Inputs=+++
  CosMy1 : Trigonometry  Operator=cos
  CosMy2 : Trigonometry  Operator=cos
  CosMy3 : Trigonometry  Operator=cos
  Gain : Gain  Gain=2/3
  Gain1 : Gain  Gain=2/3
  Product{1..6} (6 alike) : Product  RndMeth=Zero
  SinMy1 : Trigonometry
  SinMy2 : Trigonometry
  SinMy3 : Trigonometry
  Sum : Sum  Inputs=|++
  Sum1 : Sum  Inputs=++|
  nHarmonic1 : Gain
  nHarmonic2 : Gain
  phi : Constant  Value=2*pi/3
  M_tilt : Outport
  M_yaw : Outport  Port=2
  wires:
  nHarmonic2/1 -> Sum/2, CosMy1/1, SinMy1/1
  nHarmonic1/1 -> Sum1/2, Sum/1
  phi/1 -> nHarmonic1/1
  Azimuth/1 -> nHarmonic2/1
  CosMy1/1 -> Product1/2
  CosMy2/1 -> Product2/2
  SinMy1/1 -> Product4/2
  SinMy2/1 -> Product5/2
  Sum/1 -> Sum1/1, CosMy2/1, SinMy2/1
  My_1/1 -> Product4/1, Product1/1
  My_2/1 -> Product5/1, Product2/1
  Product1/1 -> Add1/1
  Product2/1 -> Add1/2
  Product4/1 -> Add2/1
  Product5/1 -> Add2/2
  Add1/1 -> Gain/1
  Add2/1 -> Gain1/1
  Sum1/1 -> SinMy3/1, CosMy3/1
  Product3/1 -> Add1/3
  My_3/1 -> Product6/1, Product3/1
  CosMy3/1 -> Product3/2
  SinMy3/1 -> Product6/2
  Product6/1 -> Add2/3
  Gain/1 -> M_tilt/1
  Gain1/1 -> M_yaw/1

== system FAST/Controller/IPC1_DataCollection/Forward Coleman Transformation 3P ==
  Azimuth : Inport
  My_1 : Inport  Port=2
  My_2 : Inport  Port=3
  My_3 : Inport  Port=4
  Add1 : Sum  Inputs=+++
  Add2 : Sum  Inputs=+++
  CosMy1 : Trigonometry  Operator=cos
  CosMy2 : Trigonometry  Operator=cos
  CosMy3 : Trigonometry  Operator=cos
  Gain : Gain  Gain=2/3
  Gain1 : Gain  Gain=2/3
  Product{1..6} (6 alike) : Product  RndMeth=Zero
  SinMy1 : Trigonometry
  SinMy2 : Trigonometry
  SinMy3 : Trigonometry
  Sum : Sum  Inputs=|++
  Sum1 : Sum  Inputs=++|
  nHarmonic : Gain  Gain=3
  nHarmonic1 : Gain  Gain=3
  phi : Constant  Value=2*pi/3
  M_tilt : Outport
  M_yaw : Outport  Port=2
  wires:
  nHarmonic1/1 -> SinMy1/1, CosMy1/1, Sum/2
  nHarmonic/1 -> Sum/1, Sum1/2
  Gain1/1 -> M_yaw/1
  Gain/1 -> M_tilt/1
  Product6/1 -> Add2/3
  SinMy3/1 -> Product6/2
  CosMy3/1 -> Product3/2
  My_3/1 -> Product3/1, Product6/1
  Product3/1 -> Add1/3
  Sum1/1 -> CosMy3/1, SinMy3/1
  Add2/1 -> Gain1/1
  Add1/1 -> Gain/1
  Product5/1 -> Add2/2
  Product4/1 -> Add2/1
  Product2/1 -> Add1/2
  Product1/1 -> Add1/1
  My_2/1 -> Product2/1, Product5/1
  My_1/1 -> Product1/1, Product4/1
  Sum/1 -> SinMy2/1, CosMy2/1, Sum1/1
  SinMy2/1 -> Product5/2
  SinMy1/1 -> Product4/2
  CosMy2/1 -> Product2/2
  CosMy1/1 -> Product1/2
  Azimuth/1 -> nHarmonic1/1
  phi/1 -> nHarmonic/1

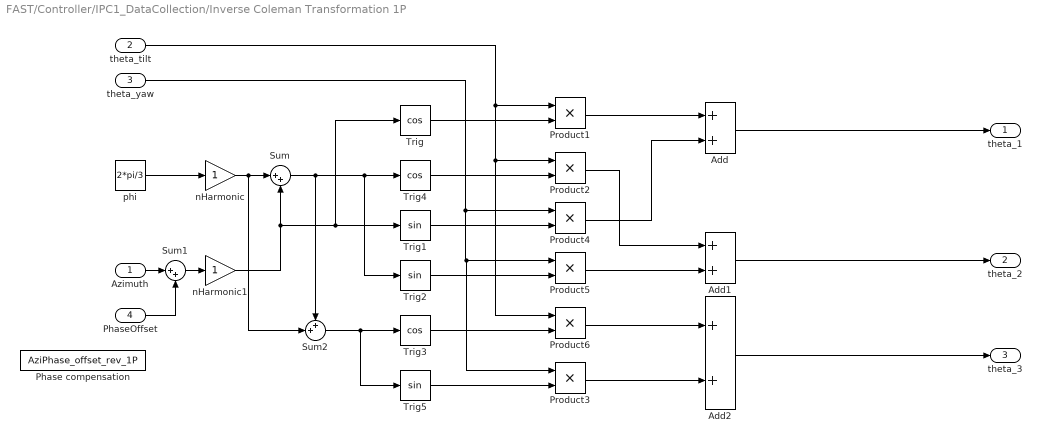
== system FAST/Controller/IPC1_DataCollection/Inverse Coleman Transformation 1P ==
  Azimuth : Inport
  theta_tilt : Inport  Port=2
  theta_yaw : Inport  Port=3
  PhaseOffset : Inport  Port=4
  Add : Sum
  Add1 : Sum
  Add2 : Sum
  Phase compensation : Constant  Value=AziPhase_offset_rev_1P
  Product{1..6} (6 alike) : Product  RndMeth=Zero
  Sum : Sum  Inputs=|++
  Sum1 : Sum  Inputs=|++
  Sum2 : Sum  Inputs=++|
  Trig : Trigonometry  Operator=cos
  Trig1 : Trigonometry
  Trig2 : Trigonometry
  Trig3 : Trigonometry  Operator=cos
  Trig4 : Trigonometry  Operator=cos
  Trig5 : Trigonometry
  nHarmonic : Gain
  nHarmonic1 : Gain
  phi : Constant  Value=2*pi/3
  theta_1 : Outport
  theta_2 : Outport  Port=2
  theta_3 : Outport  Port=3
  wires:
  Sum1/1 -> nHarmonic1/1
  Azimuth/1 -> Sum1/1
  nHarmonic/1 -> Sum/1, Sum2/2
  Add2/1 -> theta_3/1
  Add1/1 -> theta_2/1
  Add/1 -> theta_1/1
  Trig5/1 -> Product3/2
  Trig3/1 -> Product6/2
  Sum2/1 -> Trig3/1, Trig5/1
  Product3/1 -> Add2/2
  Product6/1 -> Add2/1
  PhaseOffset/1 -> Sum1/2
  Product5/1 -> Add1/2
  Product2/1 -> Add1/1
  Product1/1 -> Add/1
  Product4/1 -> Add/2
  theta_yaw/1 -> Product4/1, Product5/1, Product3/1
  theta_tilt/1 -> Product2/1, Product6/1, Product1/1
  Trig2/1 -> Product5/2
  Trig1/1 -> Product4/2
  Trig4/1 -> Product2/2
  Trig/1 -> Product1/2
  Sum/1 -> Trig2/1, Trig4/1, Sum2/1
  nHarmonic1/1 -> Sum/2, Trig1/1, Trig/1
  phi/1 -> nHarmonic/1

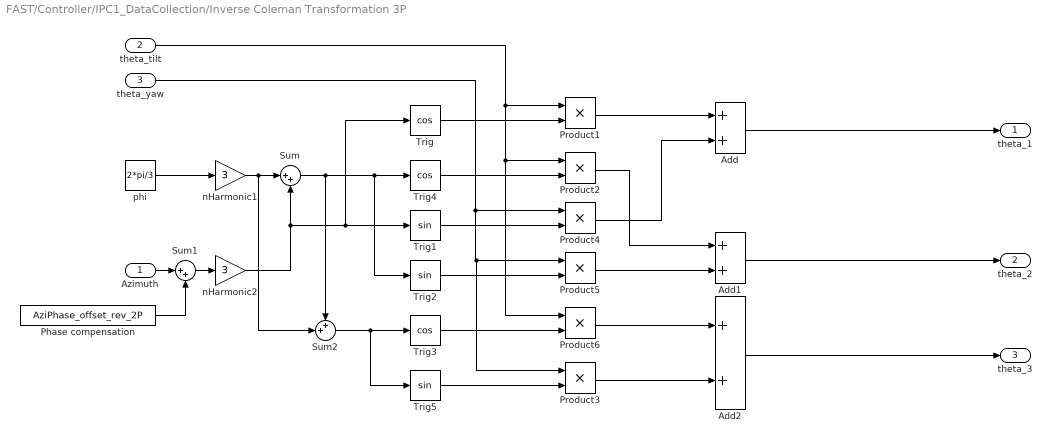
== system FAST/Controller/IPC1_DataCollection/Inverse Coleman Transformation 3P ==
  Azimuth : Inport
  theta_tilt : Inport  Port=2
  theta_yaw : Inport  Port=3
  Add : Sum
  Add1 : Sum
  Add2 : Sum
  Phase compensation : Constant  Value=AziPhase_offset_rev_2P
  Product{1..6} (6 alike) : Product  RndMeth=Zero
  Sum : Sum  Inputs=|++
  Sum1 : Sum  Inputs=|++
  Sum2 : Sum  Inputs=++|
  Trig : Trigonometry  Operator=cos
  Trig1 : Trigonometry
  Trig2 : Trigonometry
  Trig3 : Trigonometry  Operator=cos
  Trig4 : Trigonometry  Operator=cos
  Trig5 : Trigonometry
  nHarmonic1 : Gain  Gain=3
  nHarmonic2 : Gain  Gain=3
  phi : Constant  Value=2*pi/3
  theta_1 : Outport
  theta_2 : Outport  Port=2
  theta_3 : Outport  Port=3
  wires:
  nHarmonic2/1 -> Trig/1, Trig1/1, Sum/2
  Azimuth/1 -> Sum1/1
  nHarmonic1/1 -> Sum2/2, Sum/1
  phi/1 -> nHarmonic1/1
  Sum1/1 -> nHarmonic2/1
  Sum/1 -> Sum2/1, Trig4/1, Trig2/1
  Trig/1 -> Product1/2
  Trig4/1 -> Product2/2
  Trig1/1 -> Product4/2
  Trig2/1 -> Product5/2
  theta_tilt/1 -> Product1/1, Product6/1, Product2/1
  theta_yaw/1 -> Product3/1, Product5/1, Product4/1
  Product4/1 -> Add/2
  Product1/1 -> Add/1
  Product2/1 -> Add1/1
  Product5/1 -> Add1/2
  Phase compensation/1 -> Sum1/2
  Product6/1 -> Add2/1
  Product3/1 -> Add2/2
  Sum2/1 -> Trig5/1, Trig3/1
  Trig3/1 -> Product6/2
  Trig5/1 -> Product3/2
  Add/1 -> theta_1/1
  Add1/1 -> theta_2/1
  Add2/1 -> theta_3/1

== system FAST/Controller/IPC_Regulation/DiscreteTimeSSFilter1 ==
  u(k) : Inport
  A : Gain  Gain=dLP_IPC.a
  B : Gain  Gain=dLP_IPC.b
  C : Gain  Gain=dLP_IPC.c
  D : Gain  Gain=dLP_IPC.d
  Delay : Delay  DelayLength=1  InitialCondition=0
  Sum5 : Sum  Inputs=++|
  Sum6 : Sum  Inputs=++|
  y(k) : Outport
  wires:
  C/1 -> Sum6/2
  Delay/1 -> A/1, C/1
  Sum6/1 -> y(k)/1  "y(k)"
  B/1 -> Sum5/1
  D/1 -> Sum6/1
  A/1 -> Sum5/2
  u(k)/1 -> B/1, D/1
  Sum5/1 -> Delay/1

== system FAST/Controller/IPC_Regulation/DiscreteTimeSSFilter2 ==
  u(k) : Inport
  A : Gain  Gain=dLP_IPC.a
  B : Gain  Gain=dLP_IPC.b
  C : Gain  Gain=dLP_IPC.c
  D : Gain  Gain=dLP_IPC.d
  Delay : Delay  DelayLength=1  InitialCondition=0
  Sum5 : Sum  Inputs=++|
  Sum6 : Sum  Inputs=++|
  y(k) : Outport
  wires:
  Sum5/1 -> Delay/1
  u(k)/1 -> D/1, B/1
  A/1 -> Sum5/2
  D/1 -> Sum6/1
  B/1 -> Sum5/1
  Sum6/1 -> y(k)/1  "y(k)"
  Delay/1 -> C/1, A/1
  C/1 -> Sum6/2

== system FAST/Controller/IPC_Regulation/DiscreteTimeSSFilter3 ==
  u(k) : Inport
  A : Gain  Gain=dLP_IPC.a
  B : Gain  Gain=dLP_IPC.b
  C : Gain  Gain=dLP_IPC.c
  D : Gain  Gain=dLP_IPC.d
  Delay : Delay  DelayLength=1  InitialCondition=0
  Sum5 : Sum  Inputs=++|
  Sum6 : Sum  Inputs=++|
  y(k) : Outport
  wires:
  C/1 -> Sum6/2
  Delay/1 -> A/1, C/1
  Sum6/1 -> y(k)/1  "y(k)"
  B/1 -> Sum5/1
  D/1 -> Sum6/1
  A/1 -> Sum5/2
  u(k)/1 -> B/1, D/1
  Sum5/1 -> Delay/1

== system FAST/Controller/IPC_Regulation/DiscreteTimeSSFilter4 ==
  u(k) : Inport
  A : Gain  Gain=dLP.a
  B : Gain  Gain=dLP.b
  C : Gain  Gain=dLP.c
  D : Gain  Gain=dLP.d
  Delay : Delay  DelayLength=1  InitialCondition=0
  Sum5 : Sum  Inputs=++|
  Sum6 : Sum  Inputs=++|
  y(k) : Outport
  wires:
  C/1 -> Sum6/2
  Delay/1 -> A/1, C/1
  Sum6/1 -> y(k)/1  "y(k)"
  B/1 -> Sum5/1
  D/1 -> Sum6/1
  A/1 -> Sum5/2
  u(k)/1 -> B/1, D/1
  Sum5/1 -> Delay/1

== system FAST/Controller/IPC_Regulation/DiscreteTimeSSFilter5 ==
  u(k) : Inport
  A : Gain  Gain=dLP_IPC.a
  B : Gain  Gain=dLP_IPC.b
  C : Gain  Gain=dLP_IPC.c
  D : Gain  Gain=dLP_IPC.d
  Delay : Delay  DelayLength=1  InitialCondition=0
  Sum5 : Sum  Inputs=++|
  Sum6 : Sum  Inputs=++|
  y(k) : Outport
  wires:
  Sum5/1 -> Delay/1
  u(k)/1 -> D/1, B/1
  A/1 -> Sum5/2
  D/1 -> Sum6/1
  B/1 -> Sum5/1
  Sum6/1 -> y(k)/1  "y(k)"
  Delay/1 -> C/1, A/1
  C/1 -> Sum6/2
